simulink library "cjt_library_observers_compat"  (Simulink 8.7)
settings: Solver=ode45  StartTime=0.0  StopTime=10.0  RelTol=1e-3
undefined symbols (not defined in the file or in its folder): B, C, Cc, DiscIntNeverNeededParam
undefined symbols (not defined in the file): My_joint
libraries: cstblocks x4
settings Model: Creator=joern  LastModifiedBy=J�rn

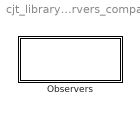
== system cjt_library_observers_compat ==
  Observers : Subsystem

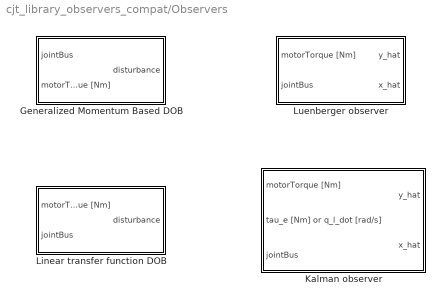
== system cjt_library_observers_compat/Observers ==
  Generalized Momentum Based DOB : Subsystem  mask(Generalized Momentum Based Disturbance Observer (DOB)){jointObj=My_joint, L=0}
      mask prompts: jointObj "Joint Object"; L "Gain L"
      mask help:
      | The observer outputs a low-pass filtered version of the actual disturbance and  introduces one parameter. The parameter is the cut-off frequency of the low-pass filter in radians/s. The observer relies on the knowledge of the joint inertia provided through the joint class.
      |
      |
      | Click >Help< for further documentation.
      mask init:
      | % Gather information about 
      | [Amat, Bmat, Cmat, Dmat, Imat, Rmat, Kmat] = rigid_gearbox(jointObj);
      | 
      | Jm = Imat(1,1);   % Effective physical inertia
      | invJm = 1/Jm;
      mask Help:
      | The block implements the generalized momentum based disturbance observer as described by Luc Le Tien  et al (2008).
      | The observer outputs a low-pass filtered version of the actual disturbance and  introduces one additional parameter. The parameter is the cut-off frequency of the low-pass filter in radians/s. The observer relies on the knowledge of the joint inertia provided through the joint class.
      | 
      | <b>Mask parameters:</b>
      | Joint Object: The class name of the CJT joint class name or the variable representing an instance of a CJT joint class.
      | Gain L: Disturbance observer gain that essentially is the cut-off frequency of a low-pass filter for the actual real disturbance given in radians/s.
      | 
      | <b>References:</b>
      | Le Tien, Luc, et al. "Friction observer and compensation for control of robots with joint torque measurement." Intelligent Robots and Systems, 2008. IROS 2008. IEEE/RSJ International Conference on. IEEE, 2008.
  Kalman observer : Subsystem  mask(Kalman estimator){jointObj=My_joint, inputIdx1_enable=on, inputIdx2_enable=off, outputIdx=[7], var_u=0.12^2, var_y=1.8e-10}
      mask prompts: jointObj "Joint Object"; inputIdx1_enable "motorTorque [Nm]"; inputIdx2_enable "tau_e [Nm] or q_l_dot [rad/s]"; outputIdx "Measured outputs (indices)"; var_u "Input noise variance(s)"; var_y "Measurement noise variance(s)"
      mask help:
      | This block implements a Kalman state estimator based on a linear state-space model of the joint. Therefore, the block relies on the function 'kalman' shipped with the Mathworks Control System Toolbox (required dependency for this block).
      |
      | Click >Help< for further documentation.
      mask init:
      | mask_Kalman_observer
      mask Help:
      | The block implements a Kalman state estimator based on a linear state-space model of the joint. Therefore, the block relies on the function 'kalman' shipped with the Mathworks Control System Toolbox (required dependency for this block).
      | 
      | <b>Mask parameters</b>
      | <b>Joint Object</b>: The class name of the CJT joint class name or the variable representing an instance of a CJT joint class.
      | <b>Measured inputs</b>: The inputs that are measured by the Kalman filter.
      | <b>Measurement Outputs</b>: vector of indices defining the elements of the output vector to be used for observation. Choices are
      | 1 - motor angle
      | 2 - gear angle
      | 3 - link  angle
      | 4 - motor velocity
      | 5 - gear velocity
      | 6  - link velocity
      | 7  - spring torque
      | 
      | <b>Input noise variance(s)</b>: Variance or variances (for multiple inputs) of the measurement noise affecting the measured inputs to the plant.
      | 
      | <b>Measurement noise variance(s)</b>: Variance or variances (for multiple outputs) of the measurement noise affecting the measured outputs to the plant.
      | 
      | <b>Notes</b>
      | For output_fixed models, when inputIdx does not contain the load velocity (input 2), it is forcibly added, as it is required for the system to be observable. Obviously during use this input can be zero for truly locked actuator outputs, but the input needs to be given to reconstruct the state of the model. See also getKalman() documentation.
      | 
      | 
      | <b>References</b>
      | [1] Franklin, G.F., J.D. Powell, and M.L. Workman, Digital Control of Dynamic Systems, Second Edition, Addison-Wesley, 1990.
      | 
      | [2] Lewis, F., Optimal Estimation, John Wiley & Sons, Inc, 1986.
      mask DialogControl Container3 Prompt: Measured inputs:
  Linear transfer function DOB : Subsystem  mask(Linear Transfer Function Disturbance Observer){loadData=off, modelFname=DOB_results.mat, jointObj=My_joint, f_c=100, measIdx=7}
      mask prompts: loadData "Load model/filters/parameters from file"; modelFname "Model/filters file (.mat)"; jointObj "Joint Object"; f_c "Q-filter cut-of frequency [Hz]"; measIdx "Measurement index"
      mask help:
      | The block implements a disturbance observer based on a linear laplace domain transfer function model of the plant.
      |
      | The block allows to select the DOB bandwidth and the joint measurement to be used. load. The joint model and  filter params can optionally chosen to to be automatically loaded from a .mat file.
      |
      | Click >Help< for further documentation.
      mask init:
      | mask_Linear_Transfer_Function_DOB
      mask Help:
      | The block implements a disturbance observer based on a linear laplace domain transfer function model of the plant as described e.g. in [1]. The implementation in this block has in particular been used to compensate plant model uncertainties and to compensate unmodelled dynamics effects in [2,3].
      | 
      | <b>Mask parameters:</b>
      | 
      | The block allows to select the DOB bandwidth and the joint measurement to be used. load. The joint model and  filter params can optionally chosen to to be automatically loaded from a .mat file.
      | 
      | Joint Object: The class name of the CJT joint class name or the variable representing an instance of a CJT joint class.
      | Q-filter cut-off frequency: Cut-off frequency  for the low-pass filter that is used to ensure causality of the observer (in Hz).
      | Measurement Index: index value that defines the element of the output vector to be used for observation. Choices are
      | 1 - motor angle
      | 2 - gear angle
      | 3 - link  angle
      | 4 - motor velocity
      | 5 - gear velocity
      | 6  - link velocity
      | 7  - spring torque
      | 
      | 
      | <b>References:</b>
      | [1] Chen, Wen-Hua, et al. "Disturbance-observer-based control and related methods—An overview." IEEE Transactions on Industrial Electronics 63.2 (2016): 1083-1095.
      | 
      | [2] Paine, Nicholas, Sehoon Oh, and Luis Sentis. "Design and control considerations for high-performance series elastic actuators." IEEE/ASME Transactions on Mechatronics 19.3 (2014): 1080-1091.
      | 
      | [3] Roozing, Wesley, et al. "Comparison of open-loop and closed-loop disturbance observers for series elastic actuators." Intelligent Robots and Systems (IROS), 2016 IEEE/RSJ International Conference on. IEEE, 2016.
      mask Callback loadData:
      | toggleMaskFields(gcbh, 'loadData', 'modelFname', 'on');
      | toggleMaskFields(gcbh, 'loadData', {'jointObj', 'f_c', 'doPlot'}, 'off');
  Luenberger observer : Subsystem  mask(Luenberger observer){jointObj=My_joint, outputIdx=[7], poles=[-100 -110 -120 -130 -140 -150]}
      mask prompts: jointObj "Joint Object"; outputIdx "Measured outputs (indices)"; poles "Observer poles"
      mask help:
      | This block implements a standard Luenberger state estimator based on a linear state-space model of the joint. Therefore, the block relies on the function 'place' shipped with the Mathworks Control System Toolbox (required dependency for this block).
      |
      | Click >Help< for further documentation.
      mask init:
      | mask_Luenberger_observer
      mask Help:
      | This block implements a standard Luenberger state estimator based on a linear state-space model of the joint. Therefore, the block relies on the function 'place' shipped with the Mathworks Control System Toolbox (required dependency for this block).
      | 
      | <b>Mask parameters</b>
      | <b>Joint Object</b>: The class name of the CJT joint class name or the variable representing an instance of a CJT joint class.
      | <b>Measurement Outputs</b>: vector of indices defining the elements of the output vector to be used for observation. Choices are
      | 1 - motor angle
      | 2 - gear angle
      | 3 - link  angle
      | 4 - motor velocity
      | 5 - gear velocity
      | 6  - link velocity
      | 7  - spring torque
      | 
      | <b>Observer poles</b>: Where to place the poles of the state observer. All poles need to be supplied, i.e. the same number as rows in the A state-space matrix of the chosen actuator model.
      | 
      | <b>References</b>
      | [1] Franklin, G.F., J.D. Powell, and M.L. Workman, Digital Control of Dynamic Systems, Second Edition, Addison-Wesley, 1990.
      | 
      | [2] Lewis, F., Optimal Estimation, John Wiley & Sons, Inc, 1986.

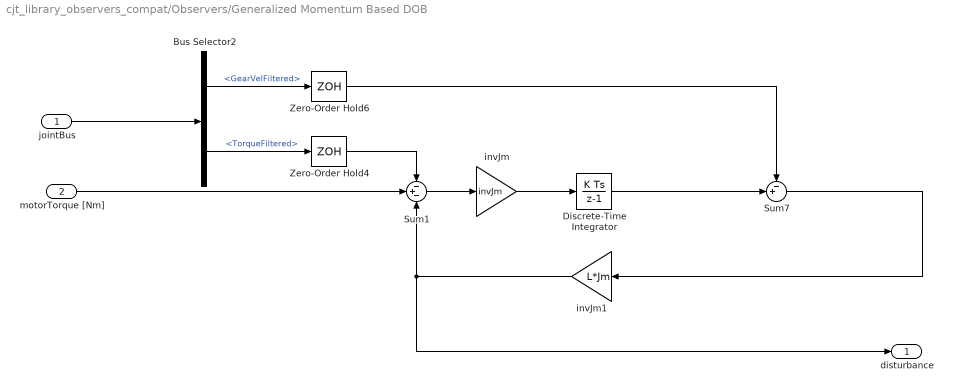
== system cjt_library_observers_compat/Observers/Generalized Momentum Based DOB ==
  jointBus : Inport
  motorTorque [Nm] : Inport  Port=2
  Bus Selector2 : BusSelector  OutputSignals=GearVelFiltered,TorqueFiltered
  Discrete-Time Integrator : DiscreteIntegrator  SampleTime=-1  ICPrevOutput=DiscIntNeverNeededParam  ICPrevScaledInput=DiscIntNeverNeededParam
  Sum1 : Sum  Inputs=-+-
  Sum7 : Sum  Inputs=-+|
  Zero-Order Hold4 : ZeroOrderHold  SampleTime=jointObj.Ts
  Zero-Order Hold6 : ZeroOrderHold  SampleTime=jointObj.Ts
  invJm : Gain  Gain=invJm
  invJm1 : Gain  Gain=L*Jm
  disturbance : Outport
  wires:
  motorTorque [Nm]/1 -> Sum1/2
  jointBus/1 -> Bus Selector2/1
  Sum7/1 -> invJm1/1
  invJm1/1 -> Sum1/3, disturbance/1
  Zero-Order Hold4/1 -> Sum1/1
  Bus Selector2/2 -> Zero-Order Hold4/1  "<TorqueFiltered>"
  Zero-Order Hold6/1 -> Sum7/1
  invJm/1 -> Discrete-Time Integrator/1
  Sum1/1 -> invJm/1
  Bus Selector2/1 -> Zero-Order Hold6/1  "<GearVelFiltered>"
  Discrete-Time Integrator/1 -> Sum7/2

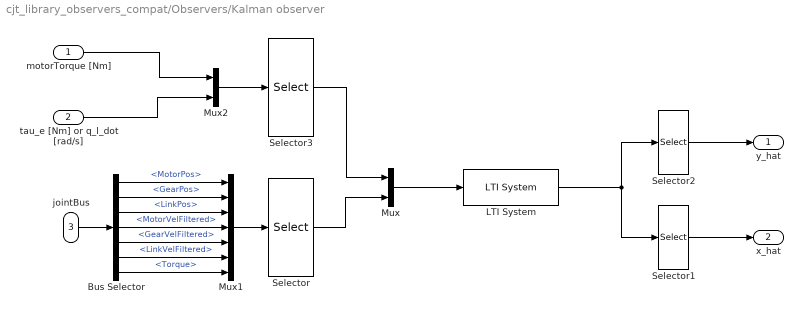
== system cjt_library_observers_compat/Observers/Kalman observer ==
  motorTorque [Nm] : Inport
  tau_e [Nm] or q_l_dot [rad/s] : Inport  Port=2
  jointBus : Inport  Port=3
  Bus Selector : BusSelector  OutputSignals=MotorPos,GearPos,LinkPos,MotorVelFiltered,GearVelFiltered,LinkVelFiltered,Torque
  LTI System : cstblocks/LTI System  sys=kest_tust  IC=[]
  Mux : Mux  Inputs=2
  Mux1 : Mux  Inputs=7
  Mux2 : Mux  Inputs=2
  Selector : Selector  InputPortWidth=size(C,1)  IndexOptions=Index vector (dialog)  Indices=outputIdx  OutputSizes=1
  Selector1 : Selector  InputPortWidth=demux_N  IndexOptions=Index vector (dialog)  Indices=demux_stateIdx  OutputSizes=1
  Selector2 : Selector  InputPortWidth=demux_N  IndexOptions=Index vector (dialog)  Indices=demux_yIdx  OutputSizes=1
  Selector3 : Selector  InputPortWidth=size(B,2)  IndexOptions=Index vector (dialog)  Indices=inputIdx  OutputSizes=1
  y_hat : Outport
  x_hat : Outport  Port=2
  wires:
  Mux/1 -> LTI System/1
  LTI System/1 -> Selector1/1, Selector2/1
  Selector1/1 -> x_hat/1
  Selector2/1 -> y_hat/1
  Selector/1 -> Mux/2
  Bus Selector/7 -> Mux1/7  "<Torque>"
  jointBus/1 -> Bus Selector/1
  Bus Selector/4 -> Mux1/4  "<MotorVelFiltered>"
  Bus Selector/2 -> Mux1/2  "<GearPos>"
  Bus Selector/6 -> Mux1/6  "<LinkVelFiltered>"
  Bus Selector/3 -> Mux1/3  "<LinkPos>"
  Bus Selector/5 -> Mux1/5  "<GearVelFiltered>"
  Bus Selector/1 -> Mux1/1  "<MotorPos>"
  Mux1/1 -> Selector/1
  Mux2/1 -> Selector3/1
  motorTorque [Nm]/1 -> Mux2/1
  tau_e [Nm] or q_l_dot [rad/s]/1 -> Mux2/2
  Selector3/1 -> Mux/1

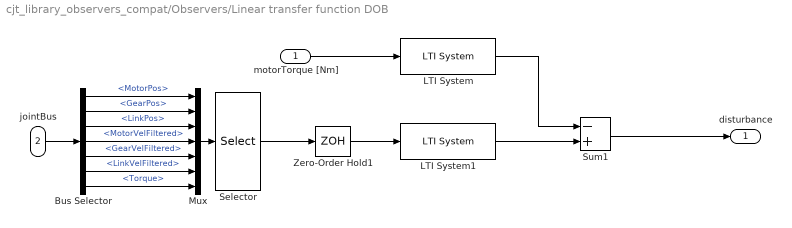
== system cjt_library_observers_compat/Observers/Linear transfer function DOB ==
  motorTorque [Nm] : Inport
  jointBus : Inport  Port=2
  Bus Selector : BusSelector  OutputSignals=MotorPos,GearPos,LinkPos,MotorVelFiltered,GearVelFiltered,LinkVelFiltered,Torque
  LTI System : cstblocks/LTI System  sys=Q_td_d  IC=[]
  LTI System1 : cstblocks/LTI System  sys=PQ_td_d  IC=[]
  Mux : Mux  Inputs=7
  Selector : Selector  InputPortWidth=size(C,1)  IndexOptions=Index vector (dialog)  Indices=measIdx  OutputSizes=1
  Sum1 : Sum  Inputs=-+
  Zero-Order Hold1 : ZeroOrderHold  SampleTime=jointObj.Ts
  disturbance : Outport
  wires:
  Zero-Order Hold1/1 -> LTI System1/1
  Bus Selector/7 -> Mux/7  "<Torque>"
  Selector/1 -> Zero-Order Hold1/1
  LTI System1/1 -> Sum1/2
  LTI System/1 -> Sum1/1
  Sum1/1 -> disturbance/1
  jointBus/1 -> Bus Selector/1
  Bus Selector/4 -> Mux/4  "<MotorVelFiltered>"
  Bus Selector/2 -> Mux/2  "<GearPos>"
  Bus Selector/6 -> Mux/6  "<LinkVelFiltered>"
  Bus Selector/3 -> Mux/3  "<LinkPos>"
  Bus Selector/5 -> Mux/5  "<GearVelFiltered>"
  Bus Selector/1 -> Mux/1  "<MotorPos>"
  Mux/1 -> Selector/1
  motorTorque [Nm]/1 -> LTI System/1

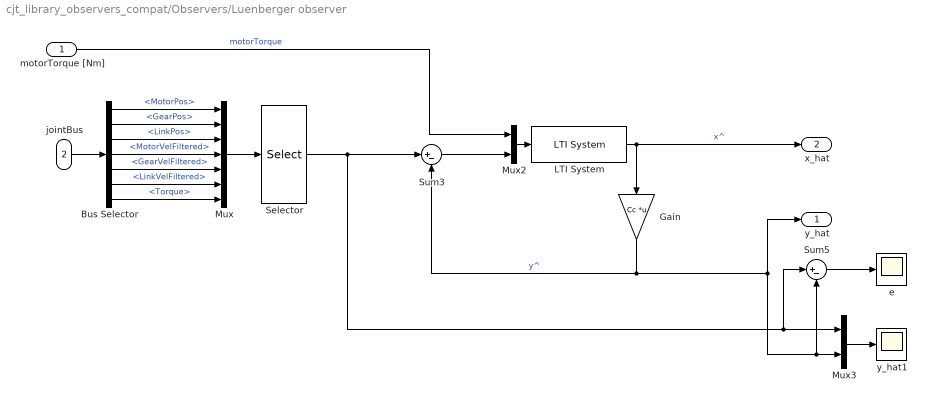
== system cjt_library_observers_compat/Observers/Luenberger observer ==
  motorTorque [Nm] : Inport
  jointBus : Inport  Port=2
  Bus Selector : BusSelector  OutputSignals=MotorPos,GearPos,LinkPos,MotorVelFiltered,GearVelFiltered,LinkVelFiltered,Torque
  Gain : Gain  Gain=Cc  Multiplication=Matrix(K*u)
  LTI System : cstblocks/LTI System  sys=sys_hat_tust  IC=[]
  Mux : Mux  Inputs=7
  Mux2 : Mux  Inputs=2
  Mux3 : Mux  Inputs=2
  Selector : Selector  InputPortWidth=size(C,1)  IndexOptions=Index vector (dialog)  Indices=outputIdx  OutputSizes=1
  Sum3 : Sum  Inputs=|+-
  Sum5 : Sum  Inputs=|+-
  e : Scope
  y_hat1 : Scope
  y_hat : Outport
  x_hat : Outport  Port=2
  wires:
  Mux3/1 -> y_hat1/1
  Sum5/1 -> e/1
  motorTorque [Nm]/1 -> Mux2/1  "motorTorque"
  LTI System/1 -> Gain/1, x_hat/1  "x^"
  Mux2/1 -> LTI System/1
  Selector/1 -> Sum3/1, Mux3/1, Sum5/1
  Sum3/1 -> Mux2/2
  Gain/1 -> y_hat/1, Sum5/2, Mux3/2, Sum3/2  "y^"
  Bus Selector/7 -> Mux/7  "<Torque>"
  jointBus/1 -> Bus Selector/1
  Bus Selector/4 -> Mux/4  "<MotorVelFiltered>"
  Bus Selector/2 -> Mux/2  "<GearPos>"
  Bus Selector/6 -> Mux/6  "<LinkVelFiltered>"
  Bus Selector/3 -> Mux/3  "<LinkPos>"
  Bus Selector/5 -> Mux/5  "<GearVelFiltered>"
  Bus Selector/1 -> Mux/1  "<MotorPos>"
  Mux/1 -> Selector/1
